simulink model "FunctionalArchitecture"  (R2022a)
settings: Solver=VariableStepAuto  StartTime=0.0  StopTime=10.0  RelTol=1e-3
settings Model: Creator=jdelolmo  LastModifiedBy=jdelolmo

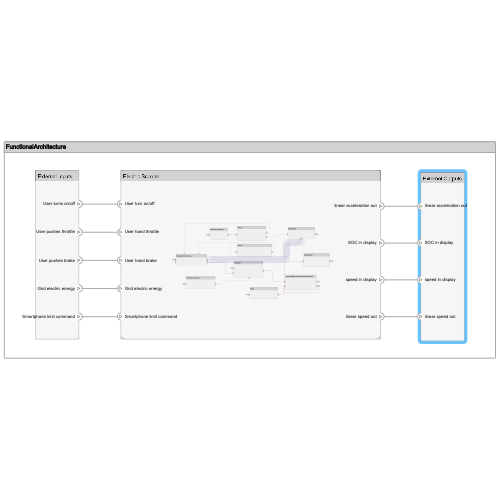
[thumbnail: Simulink's stored preview of the top-level diagram]
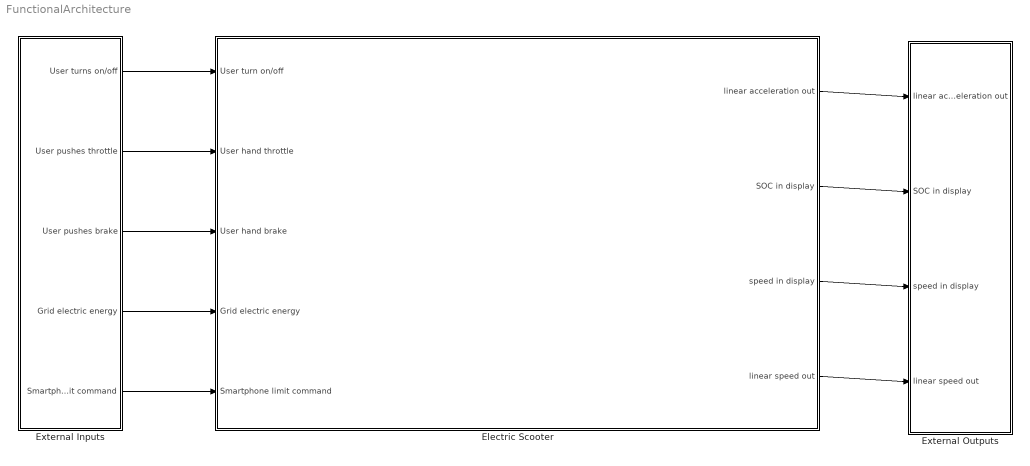
== system FunctionalArchitecture ==
  Electric Scooter : Subsystem
      settings: PortSchema="{\"entries\":[{\"content\":{\"headerSize\":26,\"margin\":15,\"minimumSpacing\":25,\"sides\":[{\"content\":{\"connectorIds\":[\"In1\",\"In2\",\"In3\",\"In4\",\"In5\"]},\"type\":\"ConnectorPlacement.EquallySpacedRectSide\",\"uuid\":\"77baa894-24de-420f-bb05-d29ca1eca7c3\"},{\"content\":{\"connectorIds\":[\"Out1\",\"Out2\",\"Out3\",\"Out4\"],\"side\":\"RIGHT\"},\"type\":\"ConnectorPlacement.EquallySpacedRectSide\",\"uuid\":\"fcd1216d-879c-477b-b249-00119a9fcd22\"},{\"content\":{\"connectorIds\":[],\"side\":\"TOP\"},\"type\":\"ConnectorPlacement.EquallySpacedRectSide\",\"uuid\":\"8485fad0-b9d7-4909-af21-eb521f98cd52\"}]},\"type\":\"ConnectorPlacement.EquallySpacedConnector\",\"uuid\":\"ff53bada-a376-4b82-92cc-106e9afccafe\"}],\"packageUris\":[\"http://schema.mathworks.com/mf0/Connector/R2020b\"],\"version\":\"1.0\"}"
  External Inputs : Subsystem
      settings: PortSchema="{\"entries\":[{\"content\":{\"headerSize\":26,\"margin\":15,\"minimumSpacing\":25,\"sides\":[{\"content\":{\"connectorIds\":[]},\"type\":\"ConnectorPlacement.EquallySpacedRectSide\",\"uuid\":\"77baa894-24de-420f-bb05-d29ca1eca7c3\"},{\"content\":{\"connectorIds\":[\"Out1\",\"Out2\",\"Out3\",\"Out4\",\"Out5\"],\"side\":\"RIGHT\"},\"type\":\"ConnectorPlacement.EquallySpacedRectSide\",\"uuid\":\"fcd1216d-879c-477b-b249-00119a9fcd22\"},{\"content\":{\"connectorIds\":[],\"side\":\"TOP\"},\"type\":\"ConnectorPlacement.EquallySpacedRectSide\",\"uuid\":\"8485fad0-b9d7-4909-af21-eb521f98cd52\"}]},\"type\":\"ConnectorPlacement.EquallySpacedConnector\",\"uuid\":\"ff53bada-a376-4b82-92cc-106e9afccafe\"}],\"packageUris\":[\"http://schema.mathworks.com/mf0/Connector/R2020b\"],\"version\":\"1.0\"}"
  External Outputs : Subsystem
      settings: PortSchema="{\"entries\":[{\"content\":{\"headerSize\":26,\"margin\":15,\"minimumSpacing\":25,\"sides\":[{\"content\":{\"connectorIds\":[\"In1\",\"In2\",\"In3\",\"In4\"]},\"type\":\"ConnectorPlacement.EquallySpacedRectSide\",\"uuid\":\"77baa894-24de-420f-bb05-d29ca1eca7c3\"},{\"content\":{\"connectorIds\":[],\"side\":\"RIGHT\"},\"type\":\"ConnectorPlacement.EquallySpacedRectSide\",\"uuid\":\"fcd1216d-879c-477b-b249-00119a9fcd22\"},{\"content\":{\"connectorIds\":[],\"side\":\"TOP\"},\"type\":\"ConnectorPlacement.EquallySpacedRectSide\",\"uuid\":\"8485fad0-b9d7-4909-af21-eb521f98cd52\"}]},\"type\":\"ConnectorPlacement.EquallySpacedConnector\",\"uuid\":\"ff53bada-a376-4b82-92cc-106e9afccafe\"}],\"packageUris\":[\"http://schema.mathworks.com/mf0/Connector/R2020b\"],\"version\":\"1.0\"}"
  wires:
  External Inputs/1(User turns on/off) -> Electric Scooter/1(User turn on/off)
  External Inputs/2(User pushes throttle) -> Electric Scooter/2(User hand throttle)
  External Inputs/3(User pushes brake) -> Electric Scooter/3(User hand brake)
  Electric Scooter/1(linear acceleration out) -> External Outputs/1(linear acceleration out)
  Electric Scooter/4(linear speed out) -> External Outputs/4(linear speed out)
  External Inputs/4(Grid electric energy) -> Electric Scooter/4(Grid electric energy)
  External Inputs/5(Smartphone limit command) -> Electric Scooter/5(Smartphone limit command)
  Electric Scooter/2(SOC in display) -> External Outputs/2(SOC in display)
  Electric Scooter/3(speed in display) -> External Outputs/3(speed in display)

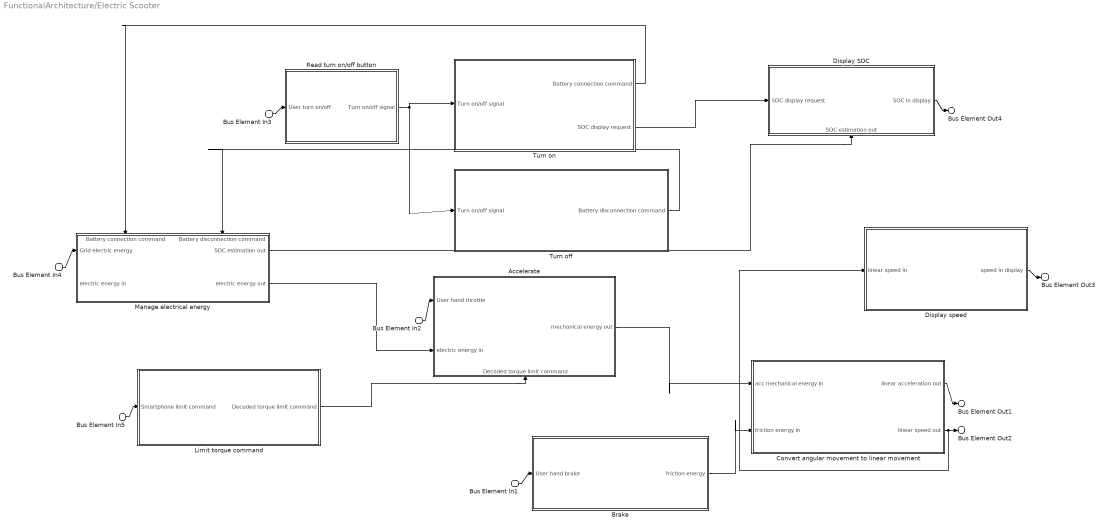
== system FunctionalArchitecture/Electric Scooter ==
  Bus Element In3 : Inport  PortName=User turn on/off
  Bus Element In2 : Inport  Port=2  PortName=User hand throttle
  Bus Element In1 : Inport  Port=3  PortName=User hand brake
  Bus Element In4 : Inport  Port=4  PortName=Grid electric energy
  Bus Element In5 : Inport  Port=5  PortName=Smartphone limit command
  Accelerate : Subsystem
      settings: PortSchema="{\"entries\":[{\"content\":{\"headerSize\":26,\"margin\":15,\"minimumSpacing\":25,\"sides\":[{\"content\":{\"connectorIds\":[\"In2\",\"In3\"]},\"type\":\"ConnectorPlacement.EquallySpacedRectSide\",\"uuid\":\"77baa894-24de-420f-bb05-d29ca1eca7c3\"},{\"content\":{\"connectorIds\":[\"Out1\"],\"side\":\"RIGHT\"},\"type\":\"ConnectorPlacement.EquallySpacedRectSide\",\"uuid\":\"fcd1216d-879c-477b-b249-00119a9fcd22\"},{\"content\":{\"connectorIds\":[],\"side\":\"TOP\"},\"type\":\"ConnectorPlacement.EquallySpacedRectSide\",\"uuid\":\"8485fad0-b9d7-4909-af21-eb521f98cd52\"},{\"content\":{\"connectorIds\":[\"In1\"],\"side\":\"BOTTOM\"},\"type\":\"ConnectorPlacement.EquallySpacedRectSide\",\"uuid\":\"51e175ef-d5f3-416f-aa43-c48a4743f776\"}]},\"type\":\"ConnectorPlacement.EquallySpacedConnector\",\"uuid\":\"ff53bada-a376-4b82-92cc-106e9afccafe\"}],\"packageUris\":[\"http://schema.mathworks.com/mf0/Connector/R2020b\"],\"version\":\"1.0\"}"
  Brake : Subsystem
      settings: PortSchema="{\"entries\":[{\"content\":{\"headerSize\":26,\"margin\":15,\"minimumSpacing\":25,\"sides\":[{\"content\":{\"connectorIds\":[\"In1\"]},\"type\":\"ConnectorPlacement.EquallySpacedRectSide\",\"uuid\":\"77baa894-24de-420f-bb05-d29ca1eca7c3\"},{\"content\":{\"connectorIds\":[\"Out1\"],\"side\":\"RIGHT\"},\"type\":\"ConnectorPlacement.EquallySpacedRectSide\",\"uuid\":\"fcd1216d-879c-477b-b249-00119a9fcd22\"},{\"content\":{\"connectorIds\":[],\"side\":\"TOP\"},\"type\":\"ConnectorPlacement.EquallySpacedRectSide\",\"uuid\":\"8485fad0-b9d7-4909-af21-eb521f98cd52\"}]},\"type\":\"ConnectorPlacement.EquallySpacedConnector\",\"uuid\":\"ff53bada-a376-4b82-92cc-106e9afccafe\"}],\"packageUris\":[\"http://schema.mathworks.com/mf0/Connector/R2020b\"],\"version\":\"1.0\"}"
  Convert angular movement to linear movement : Subsystem
      settings: PortSchema="{\"entries\":[{\"content\":{\"headerSize\":26,\"margin\":15,\"minimumSpacing\":25,\"sides\":[{\"content\":{\"connectorIds\":[\"In1\",\"In2\"]},\"type\":\"ConnectorPlacement.EquallySpacedRectSide\",\"uuid\":\"77baa894-24de-420f-bb05-d29ca1eca7c3\"},{\"content\":{\"connectorIds\":[\"Out1\",\"Out2\"],\"side\":\"RIGHT\"},\"type\":\"ConnectorPlacement.EquallySpacedRectSide\",\"uuid\":\"fcd1216d-879c-477b-b249-00119a9fcd22\"},{\"content\":{\"connectorIds\":[],\"side\":\"TOP\"},\"type\":\"ConnectorPlacement.EquallySpacedRectSide\",\"uuid\":\"8485fad0-b9d7-4909-af21-eb521f98cd52\"}]},\"type\":\"ConnectorPlacement.EquallySpacedConnector\",\"uuid\":\"ff53bada-a376-4b82-92cc-106e9afccafe\"}],\"packageUris\":[\"http://schema.mathworks.com/mf0/Connector/R2020b\"],\"version\":\"1.0\"}"
  Display SOC : Subsystem
      settings: PortSchema="{\"entries\":[{\"content\":{\"headerSize\":26,\"margin\":15,\"minimumSpacing\":25,\"sides\":[{\"content\":{\"connectorIds\":[\"In2\"]},\"type\":\"ConnectorPlacement.EquallySpacedRectSide\",\"uuid\":\"77baa894-24de-420f-bb05-d29ca1eca7c3\"},{\"content\":{\"connectorIds\":[\"Out1\"],\"side\":\"RIGHT\"},\"type\":\"ConnectorPlacement.EquallySpacedRectSide\",\"uuid\":\"fcd1216d-879c-477b-b249-00119a9fcd22\"},{\"content\":{\"connectorIds\":[],\"side\":\"TOP\"},\"type\":\"ConnectorPlacement.EquallySpacedRectSide\",\"uuid\":\"8485fad0-b9d7-4909-af21-eb521f98cd52\"},{\"content\":{\"connectorIds\":[\"In1\"],\"side\":\"BOTTOM\"},\"type\":\"ConnectorPlacement.EquallySpacedRectSide\",\"uuid\":\"2d37c353-d76b-4614-b130-29e4ea9cfd5c\"}]},\"type\":\"ConnectorPlacement.EquallySpacedConnector\",\"uuid\":\"ff53bada-a376-4b82-92cc-106e9afccafe\"}],\"packageUris\":[\"http://schema.mathworks.com/mf0/Connector/R2020b\"],\"version\":\"1.0\"}"
  Display speed : Subsystem
      settings: PortSchema="{\"entries\":[{\"content\":{\"headerSize\":26,\"margin\":15,\"minimumSpacing\":25,\"sides\":[{\"content\":{\"connectorIds\":[\"In1\"]},\"type\":\"ConnectorPlacement.EquallySpacedRectSide\",\"uuid\":\"77baa894-24de-420f-bb05-d29ca1eca7c3\"},{\"content\":{\"connectorIds\":[\"Out1\"],\"side\":\"RIGHT\"},\"type\":\"ConnectorPlacement.EquallySpacedRectSide\",\"uuid\":\"fcd1216d-879c-477b-b249-00119a9fcd22\"},{\"content\":{\"connectorIds\":[],\"side\":\"TOP\"},\"type\":\"ConnectorPlacement.EquallySpacedRectSide\",\"uuid\":\"8485fad0-b9d7-4909-af21-eb521f98cd52\"}]},\"type\":\"ConnectorPlacement.EquallySpacedConnector\",\"uuid\":\"ff53bada-a376-4b82-92cc-106e9afccafe\"}],\"packageUris\":[\"http://schema.mathworks.com/mf0/Connector/R2020b\"],\"version\":\"1.0\"}"
  Limit torque command : Subsystem
      settings: PortSchema="{\"entries\":[{\"content\":{\"headerSize\":26,\"margin\":15,\"minimumSpacing\":25,\"sides\":[{\"content\":{\"connectorIds\":[\"In1\"]},\"type\":\"ConnectorPlacement.EquallySpacedRectSide\",\"uuid\":\"77baa894-24de-420f-bb05-d29ca1eca7c3\"},{\"content\":{\"connectorIds\":[\"Out1\"],\"side\":\"RIGHT\"},\"type\":\"ConnectorPlacement.EquallySpacedRectSide\",\"uuid\":\"fcd1216d-879c-477b-b249-00119a9fcd22\"},{\"content\":{\"connectorIds\":[],\"side\":\"TOP\"},\"type\":\"ConnectorPlacement.EquallySpacedRectSide\",\"uuid\":\"8485fad0-b9d7-4909-af21-eb521f98cd52\"}]},\"type\":\"ConnectorPlacement.EquallySpacedConnector\",\"uuid\":\"ff53bada-a376-4b82-92cc-106e9afccafe\"}],\"packageUris\":[\"http://schema.mathworks.com/mf0/Connector/R2020b\"],\"version\":\"1.0\"}"
  Manage electrical energy : Subsystem
      settings: PortSchema="{\"entries\":[{\"content\":{\"headerSize\":26,\"margin\":15,\"minimumSpacing\":25,\"sides\":[{\"content\":{\"connectorIds\":[\"In3\",\"In4\"]},\"type\":\"ConnectorPlacement.EquallySpacedRectSide\",\"uuid\":\"77baa894-24de-420f-bb05-d29ca1eca7c3\"},{\"content\":{\"connectorIds\":[\"Out1\",\"Out2\"],\"side\":\"RIGHT\"},\"type\":\"ConnectorPlacement.EquallySpacedRectSide\",\"uuid\":\"fcd1216d-879c-477b-b249-00119a9fcd22\"},{\"content\":{\"connectorIds\":[\"In1\",\"In2\"],\"side\":\"TOP\"},\"type\":\"ConnectorPlacement.EquallySpacedRectSide\",\"uuid\":\"8485fad0-b9d7-4909-af21-eb521f98cd52\"}]},\"type\":\"ConnectorPlacement.EquallySpacedConnector\",\"uuid\":\"ff53bada-a376-4b82-92cc-106e9afccafe\"}],\"packageUris\":[\"http://schema.mathworks.com/mf0/Connector/R2020b\"],\"version\":\"1.0\"}"
  Read turn on/off button : Subsystem
      settings: PortSchema="{\"entries\":[{\"content\":{\"headerSize\":26,\"margin\":15,\"minimumSpacing\":25,\"sides\":[{\"content\":{\"connectorIds\":[\"In1\"]},\"type\":\"ConnectorPlacement.EquallySpacedRectSide\",\"uuid\":\"77baa894-24de-420f-bb05-d29ca1eca7c3\"},{\"content\":{\"connectorIds\":[\"Out1\"],\"side\":\"RIGHT\"},\"type\":\"ConnectorPlacement.EquallySpacedRectSide\",\"uuid\":\"fcd1216d-879c-477b-b249-00119a9fcd22\"},{\"content\":{\"connectorIds\":[],\"side\":\"TOP\"},\"type\":\"ConnectorPlacement.EquallySpacedRectSide\",\"uuid\":\"8485fad0-b9d7-4909-af21-eb521f98cd52\"}]},\"type\":\"ConnectorPlacement.EquallySpacedConnector\",\"uuid\":\"ff53bada-a376-4b82-92cc-106e9afccafe\"}],\"packageUris\":[\"http://schema.mathworks.com/mf0/Connector/R2020b\"],\"version\":\"1.0\"}"
  Turn off : Subsystem
      settings: PortSchema="{\"entries\":[{\"content\":{\"headerSize\":26,\"margin\":15,\"minimumSpacing\":25,\"sides\":[{\"content\":{\"connectorIds\":[\"In1\"]},\"type\":\"ConnectorPlacement.EquallySpacedRectSide\",\"uuid\":\"77baa894-24de-420f-bb05-d29ca1eca7c3\"},{\"content\":{\"connectorIds\":[\"Out1\"],\"side\":\"RIGHT\"},\"type\":\"ConnectorPlacement.EquallySpacedRectSide\",\"uuid\":\"fcd1216d-879c-477b-b249-00119a9fcd22\"},{\"content\":{\"connectorIds\":[],\"side\":\"TOP\"},\"type\":\"ConnectorPlacement.EquallySpacedRectSide\",\"uuid\":\"8485fad0-b9d7-4909-af21-eb521f98cd52\"}]},\"type\":\"ConnectorPlacement.EquallySpacedConnector\",\"uuid\":\"ff53bada-a376-4b82-92cc-106e9afccafe\"}],\"packageUris\":[\"http://schema.mathworks.com/mf0/Connector/R2020b\"],\"version\":\"1.0\"}"
  Turn on : Subsystem
      settings: PortSchema="{\"entries\":[{\"content\":{\"headerSize\":26,\"margin\":15,\"minimumSpacing\":25,\"sides\":[{\"content\":{\"connectorIds\":[\"In1\"]},\"type\":\"ConnectorPlacement.EquallySpacedRectSide\",\"uuid\":\"77baa894-24de-420f-bb05-d29ca1eca7c3\"},{\"content\":{\"connectorIds\":[\"Out1\",\"Out2\"],\"side\":\"RIGHT\"},\"type\":\"ConnectorPlacement.EquallySpacedRectSide\",\"uuid\":\"fcd1216d-879c-477b-b249-00119a9fcd22\"},{\"content\":{\"connectorIds\":[],\"side\":\"TOP\"},\"type\":\"ConnectorPlacement.EquallySpacedRectSide\",\"uuid\":\"8485fad0-b9d7-4909-af21-eb521f98cd52\"}]},\"type\":\"ConnectorPlacement.EquallySpacedConnector\",\"uuid\":\"ff53bada-a376-4b82-92cc-106e9afccafe\"}],\"packageUris\":[\"http://schema.mathworks.com/mf0/Connector/R2020b\"],\"version\":\"1.0\"}"
  Bus Element Out1 : Outport  PortName=linear acceleration out
  Bus Element Out4 : Outport  Port=2  PortName=SOC in display
  Bus Element Out3 : Outport  Port=3  PortName=speed in display
  Bus Element Out2 : Outport  Port=4  PortName=linear speed out
  wires:
  Bus Element In3/1 -> Read turn on/off button/1(User turn on/off)
  Read turn on/off button/1(Turn on/off signal) -> Turn off/1(Turn on/off signal), Turn on/1(Turn on/off signal)
  Bus Element In2/1 -> Accelerate/2(User hand throttle)
  Bus Element In1/1 -> Brake/1(User hand brake)
  Convert angular movement to linear movement/2(linear speed out) -> Display speed/1(linear speed in), Bus Element Out2/1
  Convert angular movement to linear movement/1(linear acceleration out) -> Bus Element Out1/1
  Accelerate/1(mechanical energy out) -> Convert angular movement to linear movement/1(acc mechanical energy in)
  Brake/1(friction energy) -> Convert angular movement to linear movement/2(friction energy in)
  Display speed/1(speed in display) -> Bus Element Out3/1
  Manage electrical energy/2(electric energy out) -> Accelerate/3(electric energy in)
  Display SOC/1(SOC in display) -> Bus Element Out4/1
  Bus Element In4/1 -> Manage electrical energy/3(Grid electric energy)
  Bus Element In5/1 -> Limit torque command/1(Smartphone limit command)
  Limit torque command/1(Decoded torque limit command) -> Accelerate/1(Decoded torque limit command)
  Turn on/1(Battery connection command) -> Manage electrical energy/1(Battery connection command)
  Turn off/1(Battery disconnection command) -> Manage electrical energy/2(Battery disconnection command)
  Turn on/2(SOC display request) -> Display SOC/2(SOC display request)
  Manage electrical energy/1(SOC estimation out) -> Display SOC/1(SOC estimation out)

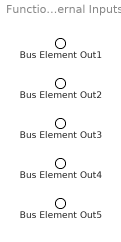
== system FunctionalArchitecture/External Inputs ==
  Bus Element Out1 : Outport  PortName=User turns on/off
  Bus Element Out2 : Outport  Port=2  PortName=User pushes throttle
  Bus Element Out3 : Outport  Port=3  PortName=User pushes brake
  Bus Element Out4 : Outport  Port=4  PortName=Grid electric energy
  Bus Element Out5 : Outport  Port=5  PortName=Smartphone limit command

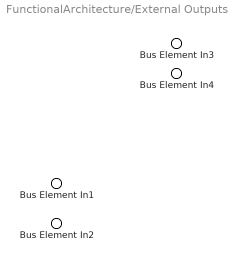
== system FunctionalArchitecture/External Outputs ==
  Bus Element In1 : Inport  PortName=linear acceleration out
  Bus Element In3 : Inport  Port=2  PortName=SOC in display
  Bus Element In4 : Inport  Port=3  PortName=speed in display
  Bus Element In2 : Inport  Port=4  PortName=linear speed out

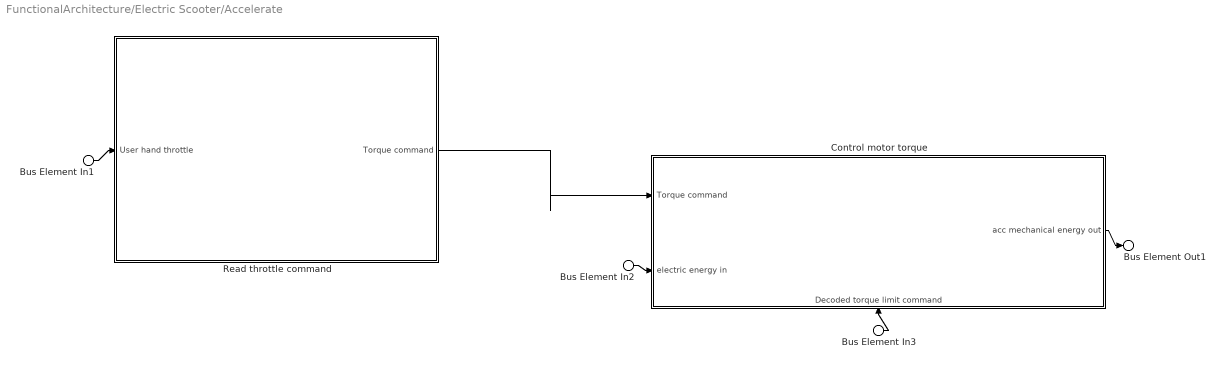
== system FunctionalArchitecture/Electric Scooter/Accelerate ==
  Bus Element In3 : Inport  PortName=Decoded torque limit command
  Bus Element In1 : Inport  Port=2  PortName=User hand throttle
  Bus Element In2 : Inport  Port=3  PortName=electric energy in
  Control motor torque : Subsystem
      settings: PortSchema="{\"entries\":[{\"content\":{\"headerSize\":26,\"margin\":15,\"minimumSpacing\":25,\"sides\":[{\"content\":{\"connectorIds\":[\"In2\",\"In3\"]},\"type\":\"ConnectorPlacement.EquallySpacedRectSide\",\"uuid\":\"77baa894-24de-420f-bb05-d29ca1eca7c3\"},{\"content\":{\"connectorIds\":[\"Out1\"],\"side\":\"RIGHT\"},\"type\":\"ConnectorPlacement.EquallySpacedRectSide\",\"uuid\":\"fcd1216d-879c-477b-b249-00119a9fcd22\"},{\"content\":{\"connectorIds\":[],\"side\":\"TOP\"},\"type\":\"ConnectorPlacement.EquallySpacedRectSide\",\"uuid\":\"8485fad0-b9d7-4909-af21-eb521f98cd52\"},{\"content\":{\"connectorIds\":[\"In1\"],\"side\":\"BOTTOM\"},\"type\":\"ConnectorPlacement.EquallySpacedRectSide\",\"uuid\":\"cc86a517-9a48-4dbd-88c6-5b6877bd718a\"}]},\"type\":\"ConnectorPlacement.EquallySpacedConnector\",\"uuid\":\"ff53bada-a376-4b82-92cc-106e9afccafe\"}],\"packageUris\":[\"http://schema.mathworks.com/mf0/Connector/R2020b\"],\"version\":\"1.0\"}"
  Read throttle command : Subsystem
      settings: PortSchema="{\"entries\":[{\"content\":{\"headerSize\":26,\"margin\":15,\"minimumSpacing\":25,\"sides\":[{\"content\":{\"connectorIds\":[\"In1\"]},\"type\":\"ConnectorPlacement.EquallySpacedRectSide\",\"uuid\":\"77baa894-24de-420f-bb05-d29ca1eca7c3\"},{\"content\":{\"connectorIds\":[\"Out1\"],\"side\":\"RIGHT\"},\"type\":\"ConnectorPlacement.EquallySpacedRectSide\",\"uuid\":\"fcd1216d-879c-477b-b249-00119a9fcd22\"},{\"content\":{\"connectorIds\":[],\"side\":\"TOP\"},\"type\":\"ConnectorPlacement.EquallySpacedRectSide\",\"uuid\":\"8485fad0-b9d7-4909-af21-eb521f98cd52\"}]},\"type\":\"ConnectorPlacement.EquallySpacedConnector\",\"uuid\":\"ff53bada-a376-4b82-92cc-106e9afccafe\"}],\"packageUris\":[\"http://schema.mathworks.com/mf0/Connector/R2020b\"],\"version\":\"1.0\"}"
  Bus Element Out1 : Outport  PortName=mechanical energy out
  wires:
  Bus Element In1/1 -> Read throttle command/1(User hand throttle)
  Read throttle command/1(Torque command) -> Control motor torque/2(Torque command)
  Control motor torque/1(acc mechanical energy out) -> Bus Element Out1/1
  Bus Element In2/1 -> Control motor torque/3(electric energy in)
  Bus Element In3/1 -> Control motor torque/1(Decoded torque limit command)

== system FunctionalArchitecture/Electric Scooter/Brake ==
  Bus Element In1 : Inport  PortName=User hand brake
  Convert mechanical energy into friction : Subsystem
      settings: PortSchema="{\"entries\":[{\"content\":{\"headerSize\":26,\"margin\":15,\"minimumSpacing\":25,\"sides\":[{\"content\":{\"connectorIds\":[\"In1\"]},\"type\":\"ConnectorPlacement.EquallySpacedRectSide\",\"uuid\":\"77baa894-24de-420f-bb05-d29ca1eca7c3\"},{\"content\":{\"connectorIds\":[\"Out1\"],\"side\":\"RIGHT\"},\"type\":\"ConnectorPlacement.EquallySpacedRectSide\",\"uuid\":\"fcd1216d-879c-477b-b249-00119a9fcd22\"},{\"content\":{\"connectorIds\":[],\"side\":\"TOP\"},\"type\":\"ConnectorPlacement.EquallySpacedRectSide\",\"uuid\":\"8485fad0-b9d7-4909-af21-eb521f98cd52\"}]},\"type\":\"ConnectorPlacement.EquallySpacedConnector\",\"uuid\":\"ff53bada-a376-4b82-92cc-106e9afccafe\"}],\"packageUris\":[\"http://schema.mathworks.com/mf0/Connector/R2020b\"],\"version\":\"1.0\"}"
  Bus Element Out1 : Outport  PortName=friction energy
  wires:
  Bus Element In1/1 -> Convert mechanical energy into friction/1(User hand brake)
  Convert mechanical energy into friction/1(friction energy) -> Bus Element Out1/1

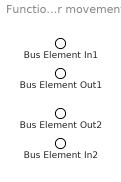
== system FunctionalArchitecture/Electric Scooter/Convert angular movement to linear movement ==
  Bus Element In1 : Inport  PortName=acc mechanical energy in
  Bus Element In2 : Inport  Port=2  PortName=friction energy in
  Bus Element Out1 : Outport  PortName=linear acceleration out
  Bus Element Out2 : Outport  Port=2  PortName=linear speed out

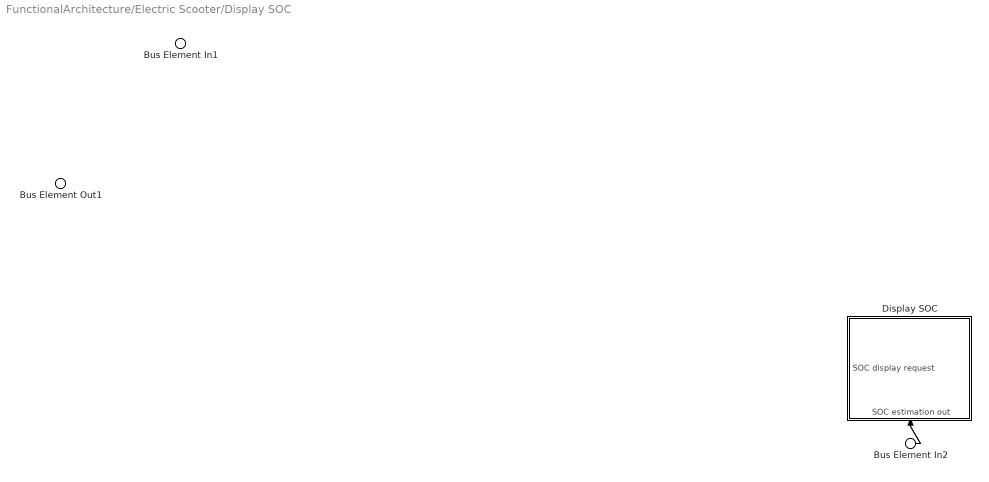
== system FunctionalArchitecture/Electric Scooter/Display SOC ==
  Bus Element In2 : Inport  PortName=SOC estimation out
  Bus Element In1 : Inport  Port=2  PortName=SOC display request
  Display SOC : Subsystem
      settings: PortSchema="{\"entries\":[{\"content\":{\"headerSize\":26,\"margin\":15,\"minimumSpacing\":25,\"sides\":[{\"content\":{\"connectorIds\":[\"In2\"]},\"type\":\"ConnectorPlacement.EquallySpacedRectSide\",\"uuid\":\"77baa894-24de-420f-bb05-d29ca1eca7c3\"},{\"content\":{\"connectorIds\":[],\"side\":\"RIGHT\"},\"type\":\"ConnectorPlacement.EquallySpacedRectSide\",\"uuid\":\"fcd1216d-879c-477b-b249-00119a9fcd22\"},{\"content\":{\"connectorIds\":[],\"side\":\"TOP\"},\"type\":\"ConnectorPlacement.EquallySpacedRectSide\",\"uuid\":\"8485fad0-b9d7-4909-af21-eb521f98cd52\"},{\"content\":{\"connectorIds\":[\"In1\"],\"side\":\"BOTTOM\"},\"type\":\"ConnectorPlacement.EquallySpacedRectSide\",\"uuid\":\"6761e298-2273-4b93-aeb1-61868e511a95\"}]},\"type\":\"ConnectorPlacement.EquallySpacedConnector\",\"uuid\":\"ff53bada-a376-4b82-92cc-106e9afccafe\"}],\"packageUris\":[\"http://schema.mathworks.com/mf0/Connector/R2020b\"],\"version\":\"1.0\"}"
  Bus Element Out1 : Outport  PortName=SOC in display
  wires:
  Bus Element In2/1 -> Display SOC/1(SOC estimation out)

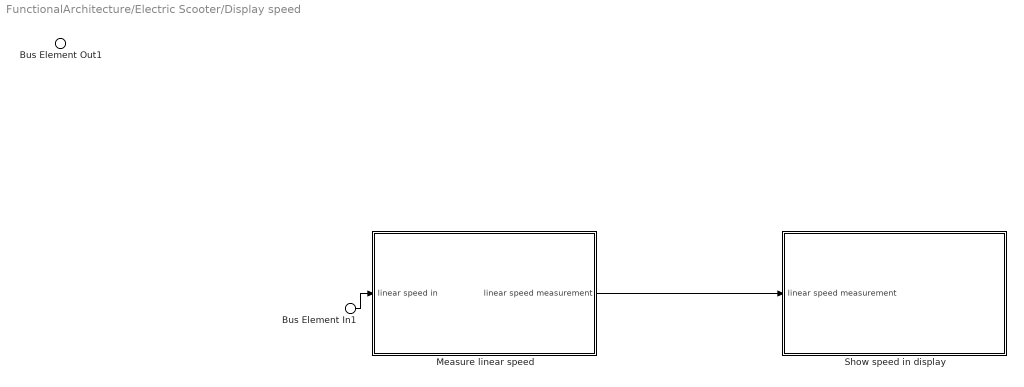
== system FunctionalArchitecture/Electric Scooter/Display speed ==
  Bus Element In1 : Inport  PortName=linear speed in
  Measure linear speed : Subsystem
      settings: PortSchema="{\"entries\":[{\"content\":{\"headerSize\":26,\"margin\":15,\"minimumSpacing\":25,\"sides\":[{\"content\":{\"connectorIds\":[\"In1\"]},\"type\":\"ConnectorPlacement.EquallySpacedRectSide\",\"uuid\":\"77baa894-24de-420f-bb05-d29ca1eca7c3\"},{\"content\":{\"connectorIds\":[\"Out1\"],\"side\":\"RIGHT\"},\"type\":\"ConnectorPlacement.EquallySpacedRectSide\",\"uuid\":\"fcd1216d-879c-477b-b249-00119a9fcd22\"},{\"content\":{\"connectorIds\":[],\"side\":\"TOP\"},\"type\":\"ConnectorPlacement.EquallySpacedRectSide\",\"uuid\":\"8485fad0-b9d7-4909-af21-eb521f98cd52\"}]},\"type\":\"ConnectorPlacement.EquallySpacedConnector\",\"uuid\":\"ff53bada-a376-4b82-92cc-106e9afccafe\"}],\"packageUris\":[\"http://schema.mathworks.com/mf0/Connector/R2020b\"],\"version\":\"1.0\"}"
  Show speed in display : Subsystem
      settings: PortSchema="{\"entries\":[{\"content\":{\"headerSize\":26,\"margin\":15,\"minimumSpacing\":25,\"sides\":[{\"content\":{\"connectorIds\":[\"In1\"]},\"type\":\"ConnectorPlacement.EquallySpacedRectSide\",\"uuid\":\"77baa894-24de-420f-bb05-d29ca1eca7c3\"},{\"content\":{\"connectorIds\":[],\"side\":\"RIGHT\"},\"type\":\"ConnectorPlacement.EquallySpacedRectSide\",\"uuid\":\"fcd1216d-879c-477b-b249-00119a9fcd22\"},{\"content\":{\"connectorIds\":[],\"side\":\"TOP\"},\"type\":\"ConnectorPlacement.EquallySpacedRectSide\",\"uuid\":\"8485fad0-b9d7-4909-af21-eb521f98cd52\"}]},\"type\":\"ConnectorPlacement.EquallySpacedConnector\",\"uuid\":\"ff53bada-a376-4b82-92cc-106e9afccafe\"}],\"packageUris\":[\"http://schema.mathworks.com/mf0/Connector/R2020b\"],\"version\":\"1.0\"}"
  Bus Element Out1 : Outport  PortName=speed in display
  wires:
  Bus Element In1/1 -> Measure linear speed/1(linear speed in)
  Measure linear speed/1(linear speed measurement) -> Show speed in display/1(linear speed measurement)

== system FunctionalArchitecture/Electric Scooter/Limit torque command ==
  Bus Element In1 : Inport  PortName=Smartphone limit command
  Decode command : Subsystem
      settings: PortSchema="{\"entries\":[{\"content\":{\"headerSize\":26,\"margin\":15,\"minimumSpacing\":25,\"sides\":[{\"content\":{\"connectorIds\":[\"In1\"]},\"type\":\"ConnectorPlacement.EquallySpacedRectSide\",\"uuid\":\"77baa894-24de-420f-bb05-d29ca1eca7c3\"},{\"content\":{\"connectorIds\":[\"Out1\"],\"side\":\"RIGHT\"},\"type\":\"ConnectorPlacement.EquallySpacedRectSide\",\"uuid\":\"fcd1216d-879c-477b-b249-00119a9fcd22\"},{\"content\":{\"connectorIds\":[],\"side\":\"TOP\"},\"type\":\"ConnectorPlacement.EquallySpacedRectSide\",\"uuid\":\"8485fad0-b9d7-4909-af21-eb521f98cd52\"}]},\"type\":\"ConnectorPlacement.EquallySpacedConnector\",\"uuid\":\"ff53bada-a376-4b82-92cc-106e9afccafe\"}],\"packageUris\":[\"http://schema.mathworks.com/mf0/Connector/R2020b\"],\"version\":\"1.0\"}"
  Bus Element Out1 : Outport  PortName=Decoded torque limit command
  wires:
  Bus Element In1/1 -> Decode command/1(Smartphone limit command)
  Decode command/1(Decoded torque limit command) -> Bus Element Out1/1

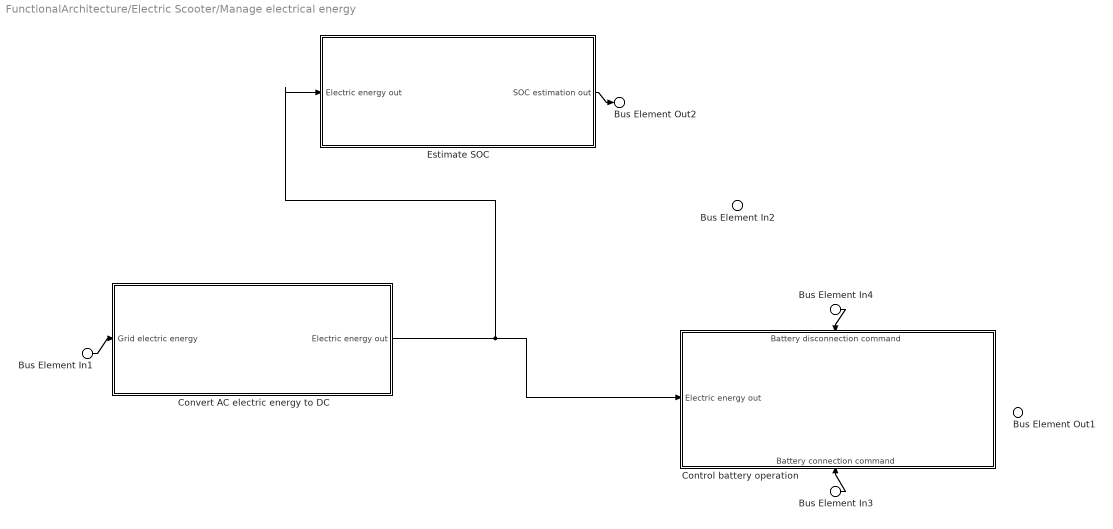
== system FunctionalArchitecture/Electric Scooter/Manage electrical energy ==
  Bus Element In3 : Inport  PortName=Battery connection command
  Bus Element In4 : Inport  Port=2  PortName=Battery disconnection command
  Bus Element In1 : Inport  Port=3  PortName=Grid electric energy
  Bus Element In2 : Inport  Port=4  PortName=electric energy in
  Control battery operation : Subsystem
      settings: PortSchema="{\"entries\":[{\"content\":{\"headerSize\":26,\"margin\":15,\"minimumSpacing\":25,\"sides\":[{\"content\":{\"connectorIds\":[\"In3\"]},\"type\":\"ConnectorPlacement.EquallySpacedRectSide\",\"uuid\":\"77baa894-24de-420f-bb05-d29ca1eca7c3\"},{\"content\":{\"connectorIds\":[],\"side\":\"RIGHT\"},\"type\":\"ConnectorPlacement.EquallySpacedRectSide\",\"uuid\":\"fcd1216d-879c-477b-b249-00119a9fcd22\"},{\"content\":{\"connectorIds\":[\"In1\"],\"side\":\"TOP\"},\"type\":\"ConnectorPlacement.EquallySpacedRectSide\",\"uuid\":\"8485fad0-b9d7-4909-af21-eb521f98cd52\"},{\"content\":{\"connectorIds\":[\"In2\"],\"side\":\"BOTTOM\"},\"type\":\"ConnectorPlacement.EquallySpacedRectSide\",\"uuid\":\"a47572cc-bc23-44f3-a706-c92f121a1f98\"}]},\"type\":\"ConnectorPlacement.EquallySpacedConnector\",\"uuid\":\"ff53bada-a376-4b82-92cc-106e9afccafe\"}],\"packageUris\":[\"http://schema.mathworks.com/mf0/Connector/R2020b\"],\"version\":\"1.0\"}"
  Convert AC electric energy to DC : Subsystem
      settings: PortSchema="{\"entries\":[{\"content\":{\"headerSize\":26,\"margin\":15,\"minimumSpacing\":25,\"sides\":[{\"content\":{\"connectorIds\":[\"In1\"]},\"type\":\"ConnectorPlacement.EquallySpacedRectSide\",\"uuid\":\"77baa894-24de-420f-bb05-d29ca1eca7c3\"},{\"content\":{\"connectorIds\":[\"Out1\"],\"side\":\"RIGHT\"},\"type\":\"ConnectorPlacement.EquallySpacedRectSide\",\"uuid\":\"fcd1216d-879c-477b-b249-00119a9fcd22\"},{\"content\":{\"connectorIds\":[],\"side\":\"TOP\"},\"type\":\"ConnectorPlacement.EquallySpacedRectSide\",\"uuid\":\"8485fad0-b9d7-4909-af21-eb521f98cd52\"}]},\"type\":\"ConnectorPlacement.EquallySpacedConnector\",\"uuid\":\"ff53bada-a376-4b82-92cc-106e9afccafe\"}],\"packageUris\":[\"http://schema.mathworks.com/mf0/Connector/R2020b\"],\"version\":\"1.0\"}"
  Estimate SOC : Subsystem
      settings: PortSchema="{\"entries\":[{\"content\":{\"headerSize\":26,\"margin\":15,\"minimumSpacing\":25,\"sides\":[{\"content\":{\"connectorIds\":[\"In1\"]},\"type\":\"ConnectorPlacement.EquallySpacedRectSide\",\"uuid\":\"77baa894-24de-420f-bb05-d29ca1eca7c3\"},{\"content\":{\"connectorIds\":[\"Out1\"],\"side\":\"RIGHT\"},\"type\":\"ConnectorPlacement.EquallySpacedRectSide\",\"uuid\":\"fcd1216d-879c-477b-b249-00119a9fcd22\"},{\"content\":{\"connectorIds\":[],\"side\":\"TOP\"},\"type\":\"ConnectorPlacement.EquallySpacedRectSide\",\"uuid\":\"8485fad0-b9d7-4909-af21-eb521f98cd52\"}]},\"type\":\"ConnectorPlacement.EquallySpacedConnector\",\"uuid\":\"ff53bada-a376-4b82-92cc-106e9afccafe\"}],\"packageUris\":[\"http://schema.mathworks.com/mf0/Connector/R2020b\"],\"version\":\"1.0\"}"
  Bus Element Out2 : Outport  PortName=SOC estimation out
  Bus Element Out1 : Outport  Port=2  PortName=electric energy out
  wires:
  Bus Element In1/1 -> Convert AC electric energy to DC/1(Grid electric energy)
  Convert AC electric energy to DC/1(Electric energy out) -> Estimate SOC/1(Electric energy out), Control battery operation/3(Electric energy out)
  Estimate SOC/1(SOC estimation out) -> Bus Element Out2/1
  Bus Element In3/1 -> Control battery operation/2(Battery connection command)
  Bus Element In4/1 -> Control battery operation/1(Battery disconnection command)

== system FunctionalArchitecture/Electric Scooter/Read turn on//off button ==
  Bus Element In1 : Inport  PortName=User turn on/off
  Bus Element Out1 : Outport  PortName=Turn on/off signal

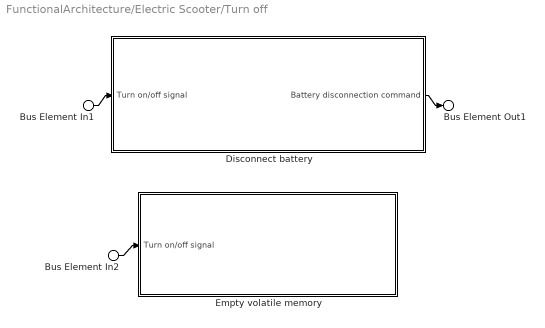
== system FunctionalArchitecture/Electric Scooter/Turn off ==
  Bus Element In1 : Inport  PortName=Turn on/off signal
  Bus Element In2 : Inport  PortName=Turn on/off signal
  Disconnect battery : Subsystem
      settings: PortSchema="{\"entries\":[{\"content\":{\"headerSize\":26,\"margin\":15,\"minimumSpacing\":25,\"sides\":[{\"content\":{\"connectorIds\":[\"In1\"]},\"type\":\"ConnectorPlacement.EquallySpacedRectSide\",\"uuid\":\"77baa894-24de-420f-bb05-d29ca1eca7c3\"},{\"content\":{\"connectorIds\":[\"Out1\"],\"side\":\"RIGHT\"},\"type\":\"ConnectorPlacement.EquallySpacedRectSide\",\"uuid\":\"fcd1216d-879c-477b-b249-00119a9fcd22\"},{\"content\":{\"connectorIds\":[],\"side\":\"TOP\"},\"type\":\"ConnectorPlacement.EquallySpacedRectSide\",\"uuid\":\"8485fad0-b9d7-4909-af21-eb521f98cd52\"}]},\"type\":\"ConnectorPlacement.EquallySpacedConnector\",\"uuid\":\"ff53bada-a376-4b82-92cc-106e9afccafe\"}],\"packageUris\":[\"http://schema.mathworks.com/mf0/Connector/R2020b\"],\"version\":\"1.0\"}"
  Empty volatile memory : Subsystem
      settings: PortSchema="{\"entries\":[{\"content\":{\"headerSize\":26,\"margin\":15,\"minimumSpacing\":25,\"sides\":[{\"content\":{\"connectorIds\":[\"In1\"]},\"type\":\"ConnectorPlacement.EquallySpacedRectSide\",\"uuid\":\"77baa894-24de-420f-bb05-d29ca1eca7c3\"},{\"content\":{\"connectorIds\":[],\"side\":\"RIGHT\"},\"type\":\"ConnectorPlacement.EquallySpacedRectSide\",\"uuid\":\"fcd1216d-879c-477b-b249-00119a9fcd22\"},{\"content\":{\"connectorIds\":[],\"side\":\"TOP\"},\"type\":\"ConnectorPlacement.EquallySpacedRectSide\",\"uuid\":\"8485fad0-b9d7-4909-af21-eb521f98cd52\"}]},\"type\":\"ConnectorPlacement.EquallySpacedConnector\",\"uuid\":\"ff53bada-a376-4b82-92cc-106e9afccafe\"}],\"packageUris\":[\"http://schema.mathworks.com/mf0/Connector/R2020b\"],\"version\":\"1.0\"}"
  Bus Element Out1 : Outport  PortName=Battery disconnection command
  wires:
  Bus Element In1/1 -> Disconnect battery/1(Turn on/off signal)
  Disconnect battery/1(Battery disconnection command) -> Bus Element Out1/1
  Bus Element In2/1 -> Empty volatile memory/1(Turn on/off signal)

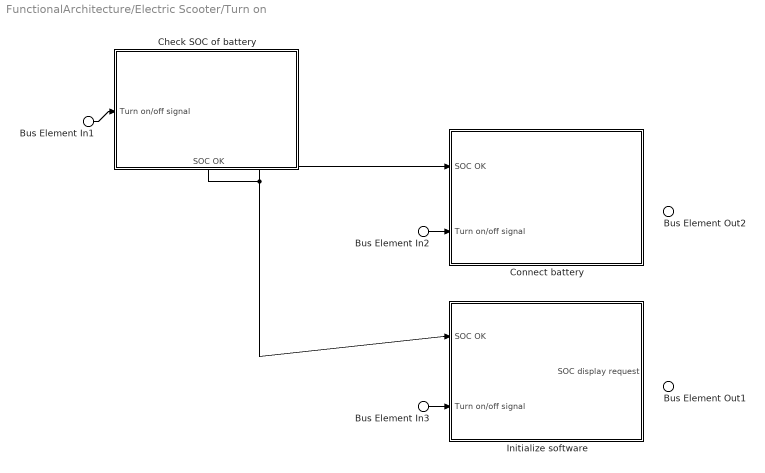
== system FunctionalArchitecture/Electric Scooter/Turn on ==
  Bus Element In1 : Inport  PortName=Turn on/off signal
  Bus Element In2 : Inport  PortName=Turn on/off signal
  Bus Element In3 : Inport  PortName=Turn on/off signal
  Check SOC of battery : Subsystem
      settings: PortSchema="{\"entries\":[{\"content\":{\"headerSize\":26,\"margin\":15,\"minimumSpacing\":25,\"sides\":[{\"content\":{\"connectorIds\":[\"In1\"]},\"type\":\"ConnectorPlacement.EquallySpacedRectSide\",\"uuid\":\"77baa894-24de-420f-bb05-d29ca1eca7c3\"},{\"content\":{\"connectorIds\":[],\"side\":\"RIGHT\"},\"type\":\"ConnectorPlacement.EquallySpacedRectSide\",\"uuid\":\"fcd1216d-879c-477b-b249-00119a9fcd22\"},{\"content\":{\"connectorIds\":[],\"side\":\"TOP\"},\"type\":\"ConnectorPlacement.EquallySpacedRectSide\",\"uuid\":\"8485fad0-b9d7-4909-af21-eb521f98cd52\"},{\"content\":{\"connectorIds\":[\"Out1\"],\"side\":\"BOTTOM\"},\"type\":\"ConnectorPlacement.EquallySpacedRectSide\",\"uuid\":\"1b52d42d-0e9e-4274-b6a6-d9e1a3e227e2\"}]},\"type\":\"ConnectorPlacement.EquallySpacedConnector\",\"uuid\":\"ff53bada-a376-4b82-92cc-106e9afccafe\"}],\"packageUris\":[\"http://schema.mathworks.com/mf0/Connector/R2020b\"],\"version\":\"1.0\"}"
  Connect battery : Subsystem
      settings: PortSchema="{\"entries\":[{\"content\":{\"headerSize\":26,\"margin\":15,\"minimumSpacing\":25,\"sides\":[{\"content\":{\"connectorIds\":[\"In1\",\"In2\"]},\"type\":\"ConnectorPlacement.EquallySpacedRectSide\",\"uuid\":\"77baa894-24de-420f-bb05-d29ca1eca7c3\"},{\"content\":{\"connectorIds\":[],\"side\":\"RIGHT\"},\"type\":\"ConnectorPlacement.EquallySpacedRectSide\",\"uuid\":\"fcd1216d-879c-477b-b249-00119a9fcd22\"},{\"content\":{\"connectorIds\":[],\"side\":\"TOP\"},\"type\":\"ConnectorPlacement.EquallySpacedRectSide\",\"uuid\":\"8485fad0-b9d7-4909-af21-eb521f98cd52\"}]},\"type\":\"ConnectorPlacement.EquallySpacedConnector\",\"uuid\":\"ff53bada-a376-4b82-92cc-106e9afccafe\"}],\"packageUris\":[\"http://schema.mathworks.com/mf0/Connector/R2020b\"],\"version\":\"1.0\"}"
  Initialize software : Subsystem
      settings: PortSchema="{\"entries\":[{\"content\":{\"headerSize\":26,\"margin\":15,\"minimumSpacing\":25,\"sides\":[{\"content\":{\"connectorIds\":[\"In1\",\"In2\"]},\"type\":\"ConnectorPlacement.EquallySpacedRectSide\",\"uuid\":\"77baa894-24de-420f-bb05-d29ca1eca7c3\"},{\"content\":{\"connectorIds\":[\"Out1\"],\"side\":\"RIGHT\"},\"type\":\"ConnectorPlacement.EquallySpacedRectSide\",\"uuid\":\"fcd1216d-879c-477b-b249-00119a9fcd22\"},{\"content\":{\"connectorIds\":[],\"side\":\"TOP\"},\"type\":\"ConnectorPlacement.EquallySpacedRectSide\",\"uuid\":\"8485fad0-b9d7-4909-af21-eb521f98cd52\"}]},\"type\":\"ConnectorPlacement.EquallySpacedConnector\",\"uuid\":\"ff53bada-a376-4b82-92cc-106e9afccafe\"}],\"packageUris\":[\"http://schema.mathworks.com/mf0/Connector/R2020b\"],\"version\":\"1.0\"}"
  Bus Element Out2 : Outport  PortName=Battery connection command
  Bus Element Out1 : Outport  Port=2  PortName=SOC display request
  wires:
  Check SOC of battery/1(SOC OK) -> Initialize software/1(SOC OK), Connect battery/1(SOC OK)
  Bus Element In1/1 -> Check SOC of battery/1(Turn on/off signal)
  Bus Element In2/1 -> Connect battery/2(Turn on/off signal)
  Bus Element In3/1 -> Initialize software/2(Turn on/off signal)

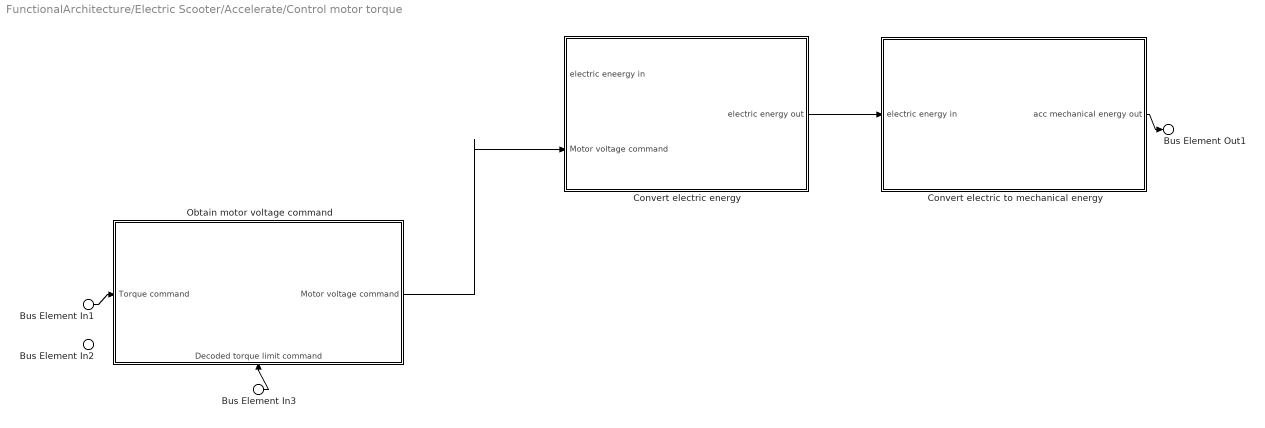
== system FunctionalArchitecture/Electric Scooter/Accelerate/Control motor torque ==
  Bus Element In3 : Inport  PortName=Decoded torque limit command
  Bus Element In1 : Inport  Port=2  PortName=Torque command
  Bus Element In2 : Inport  Port=3  PortName=electric energy in
  Convert electric energy : Subsystem
      settings: PortSchema="{\"entries\":[{\"content\":{\"headerSize\":26,\"margin\":15,\"minimumSpacing\":25,\"sides\":[{\"content\":{\"connectorIds\":[\"In1\",\"In2\"]},\"type\":\"ConnectorPlacement.EquallySpacedRectSide\",\"uuid\":\"77baa894-24de-420f-bb05-d29ca1eca7c3\"},{\"content\":{\"connectorIds\":[\"Out1\"],\"side\":\"RIGHT\"},\"type\":\"ConnectorPlacement.EquallySpacedRectSide\",\"uuid\":\"fcd1216d-879c-477b-b249-00119a9fcd22\"},{\"content\":{\"connectorIds\":[],\"side\":\"TOP\"},\"type\":\"ConnectorPlacement.EquallySpacedRectSide\",\"uuid\":\"8485fad0-b9d7-4909-af21-eb521f98cd52\"}]},\"type\":\"ConnectorPlacement.EquallySpacedConnector\",\"uuid\":\"ff53bada-a376-4b82-92cc-106e9afccafe\"}],\"packageUris\":[\"http://schema.mathworks.com/mf0/Connector/R2020b\"],\"version\":\"1.0\"}"
  Convert electric to mechanical energy : Subsystem
      settings: PortSchema="{\"entries\":[{\"content\":{\"headerSize\":26,\"margin\":15,\"minimumSpacing\":25,\"sides\":[{\"content\":{\"connectorIds\":[\"In1\"]},\"type\":\"ConnectorPlacement.EquallySpacedRectSide\",\"uuid\":\"77baa894-24de-420f-bb05-d29ca1eca7c3\"},{\"content\":{\"connectorIds\":[\"Out1\"],\"side\":\"RIGHT\"},\"type\":\"ConnectorPlacement.EquallySpacedRectSide\",\"uuid\":\"fcd1216d-879c-477b-b249-00119a9fcd22\"},{\"content\":{\"connectorIds\":[],\"side\":\"TOP\"},\"type\":\"ConnectorPlacement.EquallySpacedRectSide\",\"uuid\":\"8485fad0-b9d7-4909-af21-eb521f98cd52\"},{\"content\":{\"connectorIds\":[],\"side\":\"BOTTOM\"},\"type\":\"ConnectorPlacement.EquallySpacedRectSide\",\"uuid\":\"90bb9375-eb9b-40f0-ae23-8bb920906b4a\"}]},\"type\":\"ConnectorPlacement.EquallySpacedConnector\",\"uuid\":\"ff53bada-a376-4b82-92cc-106e9afccafe\"}],\"packageUris\":[\"http://schema.mathworks.com/mf0/Connector/R2020b\"],\"version\":\"1.0\"}"
  Obtain motor voltage command : Subsystem
      settings: PortSchema="{\"entries\":[{\"content\":{\"headerSize\":26,\"margin\":15,\"minimumSpacing\":25,\"sides\":[{\"content\":{\"connectorIds\":[\"In2\"]},\"type\":\"ConnectorPlacement.EquallySpacedRectSide\",\"uuid\":\"77baa894-24de-420f-bb05-d29ca1eca7c3\"},{\"content\":{\"connectorIds\":[\"Out1\"],\"side\":\"RIGHT\"},\"type\":\"ConnectorPlacement.EquallySpacedRectSide\",\"uuid\":\"fcd1216d-879c-477b-b249-00119a9fcd22\"},{\"content\":{\"connectorIds\":[],\"side\":\"TOP\"},\"type\":\"ConnectorPlacement.EquallySpacedRectSide\",\"uuid\":\"8485fad0-b9d7-4909-af21-eb521f98cd52\"},{\"content\":{\"connectorIds\":[\"In1\"],\"side\":\"BOTTOM\"},\"type\":\"ConnectorPlacement.EquallySpacedRectSide\",\"uuid\":\"a45a436b-2e63-4e58-a9ce-9fd992ea0ca5\"}]},\"type\":\"ConnectorPlacement.EquallySpacedConnector\",\"uuid\":\"ff53bada-a376-4b82-92cc-106e9afccafe\"}],\"packageUris\":[\"http://schema.mathworks.com/mf0/Connector/R2020b\"],\"version\":\"1.0\"}"
  Bus Element Out1 : Outport  PortName=acc mechanical energy out
  wires:
  Bus Element In1/1 -> Obtain motor voltage command/2(Torque command)
  Obtain motor voltage command/1(Motor voltage command) -> Convert electric energy/2(Motor voltage command)
  Convert electric energy/1(electric energy out) -> Convert electric to mechanical energy/1(electric energy in)
  Convert electric to mechanical energy/1(acc mechanical energy out) -> Bus Element Out1/1
  Bus Element In3/1 -> Obtain motor voltage command/1(Decoded torque limit command)

== system FunctionalArchitecture/Electric Scooter/Accelerate/Read throttle command ==
  Bus Element In1 : Inport  PortName=User hand throttle
  Bus Element Out1 : Outport  PortName=Torque command

== system FunctionalArchitecture/Electric Scooter/Brake/Convert mechanical energy into friction ==
  Bus Element In1 : Inport  PortName=User hand brake
  Bus Element Out1 : Outport  PortName=friction energy

== system FunctionalArchitecture/Electric Scooter/Display SOC/Display SOC ==
  Bus Element In2 : Inport  PortName=SOC estimation out
  Bus Element In1 : Inport  Port=2  PortName=SOC display request

== system FunctionalArchitecture/Electric Scooter/Display speed/Measure linear speed ==
  Bus Element In1 : Inport  PortName=linear speed in
  Bus Element Out1 : Outport  PortName=linear speed measurement

== system FunctionalArchitecture/Electric Scooter/Display speed/Show speed in display ==
  Bus Element In1 : Inport  PortName=linear speed measurement

== system FunctionalArchitecture/Electric Scooter/Limit torque command/Decode command ==
  Bus Element In1 : Inport  PortName=Smartphone limit command
  Bus Element Out1 : Outport  PortName=Decoded torque limit command

== system FunctionalArchitecture/Electric Scooter/Manage electrical energy/Control battery operation ==
  Bus Element In3 : Inport  PortName=Battery disconnection command
  Bus Element In2 : Inport  Port=2  PortName=Battery connection command
  Bus Element In1 : Inport  Port=3  PortName=Electric energy out

== system FunctionalArchitecture/Electric Scooter/Manage electrical energy/Convert AC electric energy to DC ==
  Bus Element In1 : Inport  PortName=Grid electric energy
  Bus Element Out1 : Outport  PortName=Electric energy out

== system FunctionalArchitecture/Electric Scooter/Manage electrical energy/Estimate SOC ==
  Bus Element In1 : Inport  PortName=Electric energy out
  Bus Element Out1 : Outport  PortName=SOC estimation out

== system FunctionalArchitecture/Electric Scooter/Turn off/Disconnect battery ==
  Bus Element In1 : Inport  PortName=Turn on/off signal
  Bus Element Out1 : Outport  PortName=Battery disconnection command

== system FunctionalArchitecture/Electric Scooter/Turn off/Empty volatile memory ==
  Bus Element In1 : Inport  PortName=Turn on/off signal

== system FunctionalArchitecture/Electric Scooter/Turn on/Check SOC of battery ==
  Bus Element In1 : Inport  PortName=Turn on/off signal
  Bus Element Out1 : Outport  PortName=SOC OK

== system FunctionalArchitecture/Electric Scooter/Turn on/Connect battery ==
  Bus Element In1 : Inport  PortName=SOC OK
  Bus Element In2 : Inport  Port=2  PortName=Turn on/off signal

== system FunctionalArchitecture/Electric Scooter/Turn on/Initialize software ==
  Bus Element In2 : Inport  PortName=SOC OK
  Bus Element In1 : Inport  Port=2  PortName=Turn on/off signal
  Bus Element Out1 : Outport  PortName=SOC display request

== system FunctionalArchitecture/Electric Scooter/Accelerate/Control motor torque/Convert electric energy ==
  Bus Element In2 : Inport  PortName=electric eneergy in
  Bus Element In1 : Inport  Port=2  PortName=Motor voltage command
  Bus Element Out1 : Outport  PortName=electric energy out

== system FunctionalArchitecture/Electric Scooter/Accelerate/Control motor torque/Convert electric to mechanical energy ==
  Bus Element In1 : Inport  PortName=electric energy in
  Bus Element Out1 : Outport  PortName=acc mechanical energy out

== system FunctionalArchitecture/Electric Scooter/Accelerate/Control motor torque/Obtain motor voltage command ==
  Bus Element In2 : Inport  PortName=Decoded torque limit command
  Bus Element In1 : Inport  Port=2  PortName=Torque command
  Bus Element Out1 : Outport  PortName=Motor voltage command
